simulink model "park"  (R2016a)
settings: Solver=VariableStepAuto  StartTime=0.0  StopTime=10.0  RelTol=1e-3
settings Model: Creator=rtw141  LastModifiedBy=rtw141
settings GRTTargetCC: GeneratePreprocessorConditionals=Use local settings

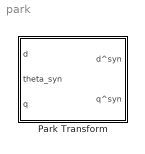
== system park ==
  Park Transform : Subsystem

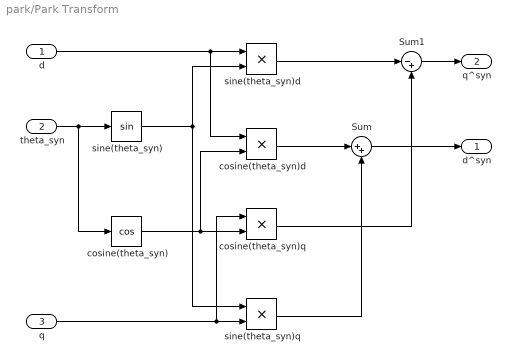
== system park/Park Transform ==
  d : Inport
  theta_syn : Inport  Port=2
  q : Inport  Port=3
  Sum : Sum  Inputs=|++
  Sum1 : Sum  Inputs=|-+
  cosine(theta_syn) : Trigonometry  Operator=cos
  cosine(theta_syn)d : Product
  cosine(theta_syn)q : Product
  sine(theta_syn) : Trigonometry
  sine(theta_syn)d : Product
  sine(theta_syn)q : Product
  d^syn : Outport
  q^syn : Outport  Port=2
  wires:
  Sum1/1 -> q^syn/1
  cosine(theta_syn)q/1 -> Sum1/2
  cosine(theta_syn)d/1 -> Sum/1
  q/1 -> cosine(theta_syn)q/1, sine(theta_syn)q/2
  sine(theta_syn)q/1 -> Sum/2
  cosine(theta_syn)/1 -> cosine(theta_syn)q/2, cosine(theta_syn)d/2
  Sum/1 -> d^syn/1
  sine(theta_syn)d/1 -> Sum1/1
  theta_syn/1 -> cosine(theta_syn)/1, sine(theta_syn)/1
  d/1 -> cosine(theta_syn)d/1, sine(theta_syn)d/1
  sine(theta_syn)/1 -> sine(theta_syn)q/1, sine(theta_syn)d/2
